simulink model "chap7_12sim"  (Simulink 5.0)
settings: Solver=ode45  StartTime=0.0  StopTime=2  RelTol=1e-3
settings Model: LastModifiedBy=Administrator

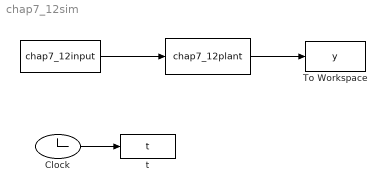
== system chap7_12sim ==
  " " : S-Function  FunctionName=chap7_12input
  "  " : S-Function  FunctionName=chap7_12plant
  Clock : Clock
      settings: Decimation=10
  To Workspace : ToWorkspace  VariableName=y  SampleTime=-1  SaveFormat=Array
  t : ToWorkspace  VariableName=t  SampleTime=-1  SaveFormat=Array
  wires:
  "  "/1 -> To Workspace/1
  Clock/1 -> t/1
  " "/1 -> "  "/1
